simulink model "RC_filter_system"  (R2018b)
settings: Solver=FixedStepAuto  StartTime=0.0  StopTime=100  FixedStep=0.001  RelTol=1e-3
InitFcn:
  | Parameters
values from neighbouring files (symbols this model uses):
  tau = R*C    (= 0.1113767)    [Parameters.m]
settings Model: Creator=alessandrosebastianelli  LastModifiedBy=alessandrosebastianelli

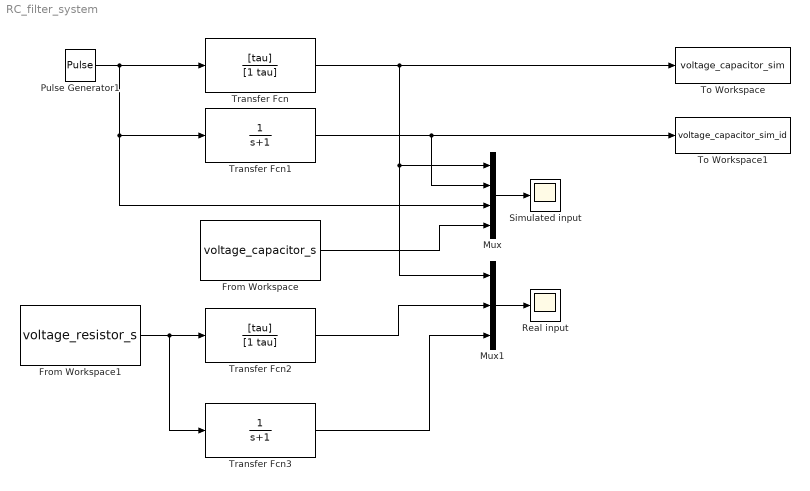
== system RC_filter_system ==
  From Workspace : FromWorkspace  VariableName=voltage_capacitor_s  SampleTime=0.001
  From Workspace1 : FromWorkspace  VariableName=voltage_resistor_s  SampleTime=0.001
  Mux : Mux
  Mux1 : Mux  Inputs=3
  Pulse Generator1 : DiscretePulseGenerator  PulseType=Time based  Amplitude=5  Period=30  PulseWidth=50  SampleTime=-1
  "Real input " : Scope
  "Simulated input " : Scope
  To Workspace : ToWorkspace  VariableName=voltage_capacitor_sim  SaveFormat=Timeseries  SampleTime=-1
      settings: Save2DSignal=2-D array (concatenate along first dimension)
  To Workspace1 : ToWorkspace  VariableName=voltage_capacitor_sim_id  SaveFormat=Timeseries  SampleTime=-1
      settings: Save2DSignal=2-D array (concatenate along first dimension)
  Transfer Fcn : TransferFcn  Numerator=[tau]  Denominator=[1 tau]
  Transfer Fcn1 : TransferFcn  Denominator=[1 1]
  Transfer Fcn2 : TransferFcn  Numerator=[tau]  Denominator=[1 tau]
  Transfer Fcn3 : TransferFcn  Denominator=[1 1]
  wires:
  Pulse Generator1/1 -> Mux/3, Transfer Fcn1/1, Transfer Fcn/1
  Transfer Fcn/1 -> To Workspace/1, Mux1/1, Mux/1
  From Workspace/1 -> Mux/4
  Mux/1 -> "Simulated input "/1
  Transfer Fcn1/1 -> Mux/2, To Workspace1/1
  From Workspace1/1 -> Transfer Fcn3/1, Transfer Fcn2/1
  Transfer Fcn2/1 -> Mux1/2
  Mux1/1 -> "Real input "/1
  Transfer Fcn3/1 -> Mux1/3
